simulink model "ballcl"  (R2017a)
settings: Solver=ode45  StartTime=0.0  StopTime=10.0  RelTol=1e-3
values from neighbouring files (symbols this model uses):
  d = 0.1    [BallAndBeamSystemTest.m]
  g = -9.8    [BallAndBeamSystemTest.m]
  J = 1.416e-4    (= 0.0001416)    [BallAndBeamSystemTest.m]
  L = 1.0    (= 1)    [BallAndBeamSystemTest.m]
  m = 0.220    (= 0.22)    [BallAndBeamSystemTest.m]
  R = 0.04    [BallAndBeamSystemTest.m]
settings Model: Creator=sansh  LastModifiedBy=sansh

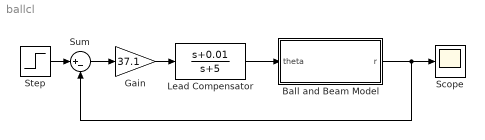
== system ballcl ==
  Ball and Beam Model : Subsystem
  Gain : Gain  Gain=37.1
  Lead Compensator : TransferFcn  Numerator=[1 0.01]  Denominator=[1 5]
  Scope : Scope
  Step : Step  Time=0  SampleTime=0
  Sum : Sum  Inputs=|+-
  wires:
  Ball and Beam Model/1(r) -> Sum/2, Scope/1
  Lead Compensator/1 -> Ball and Beam Model/1(theta)
  Gain/1 -> Lead Compensator/1
  Step/1 -> Sum/1
  Sum/1 -> Gain/1

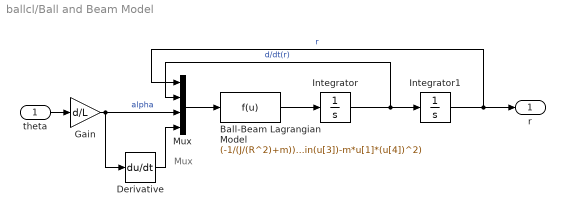
== system ballcl/Ball and Beam Model ==
  note: Mux
  theta : Inport
  Ball-Beam Lagrangian Model : Fcn  Expr=(-1/(J/(R^2)+m))*(m*g*sin(u[3])-m*u[1]*(u[4])^2)
  Derivative : Derivative
  Gain : Gain  Gain=d/L
  Integrator : Integrator
  Integrator1 : Integrator
  Mux : Mux
  r : Outport
  wires:
  theta/1 -> Gain/1
  Gain/1 -> Derivative/1, Mux/3  "alpha"
  Ball-Beam Lagrangian Model/1 -> Integrator/1
  Derivative/1 -> Mux/4
  Integrator1/1 -> Mux/1, r/1  "r"
  Mux/1 -> Ball-Beam Lagrangian Model/1
  Integrator/1 -> Mux/2, Integrator1/1  "d/dt(r)"
